simulink model "rocket3"  (R2012b)
settings: Solver=ode3  StartTime=0  StopTime=5  FixedStep=0.0005  RelTol=1e-3
undefined symbols (not defined in the file): dfilt, DiscIntNeverNeededParam, fdesignblkfcn, gcbh
libraries: mblibv1 x17, simulink x1, dsparch4 x1
settings Model: BufferReuse=off  Creator=David  LastModifiedBy=David
settings OptimizationCC: InlineParams=on  BufferReuse=off  SimCompilerOptimization=On
settings DebuggingCC: InitInArrayFormatMsg=none
settings SimMechanicsCC: VisDuringSimulation=on
settings ConfigurationSet: Description=SimMechanics 2G

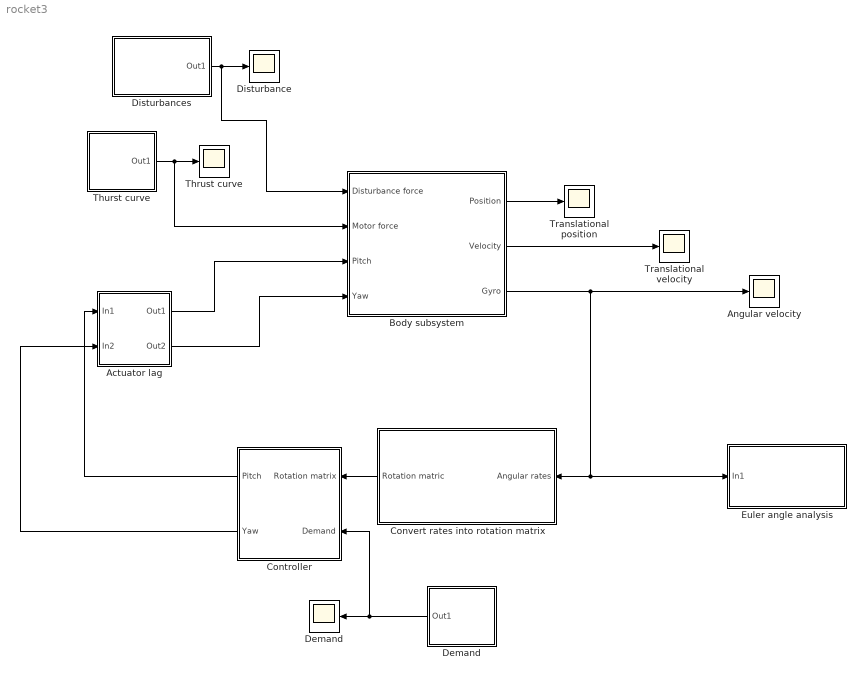
== system rocket3 ==
  Actuator lag : Subsystem
  Angular velocity : Scope
      settings: ShowLegends=on  YMin=-2.5  YMax=0  SaveName=ScopeData2
  Body subsystem : Subsystem
  "Controller " : Subsystem
  Convert rates into rotation matrix : Subsystem
  Demand : Subsystem
  "Demand " : Scope
      settings: YMin=-0.1  YMax=0.09  SaveName=ScopeData8  SampleTime=5
  Disturbance : Scope
      settings: YMin=-0.1  YMax=0.09  SaveName=ScopeData10  SampleTime=5
  Disturbances : Subsystem
  Euler angle analysis : Subsystem
  Thrust curve : Scope
      settings: YMin=-0.1  YMax=0.09  SaveName=ScopeData7
  "Thurst curve " : Subsystem
  Translational position : Scope
      settings: ShowLegends=on
  Translational velocity : Scope
  wires:
  Body subsystem/1(Position) -> Translational position/1
  Body subsystem/2(Velocity) -> Translational velocity/1
  Body subsystem/3(Gyro) -> Angular velocity/1, Euler angle analysis/1(In1), Convert rates into rotation matrix/1(Angular rates)
  Disturbances/1(Out1) -> Body subsystem/1(Disturbance force), Disturbance/1
  "Thurst curve "/1(Out1) -> Body subsystem/2(Motor force), Thrust curve/1
  Convert rates into rotation matrix/1(Rotation matric) -> "Controller "/1(Rotation matrix)
  Demand/1(Out1) -> "Demand "/1, "Controller "/2(Demand)
  "Controller "/1(Pitch) -> Actuator lag/1(In1)
  "Controller "/2(Yaw) -> Actuator lag/2(In2)
  Actuator lag/1(Out1) -> Body subsystem/3(Pitch)
  Actuator lag/2(Out2) -> Body subsystem/4(Yaw)

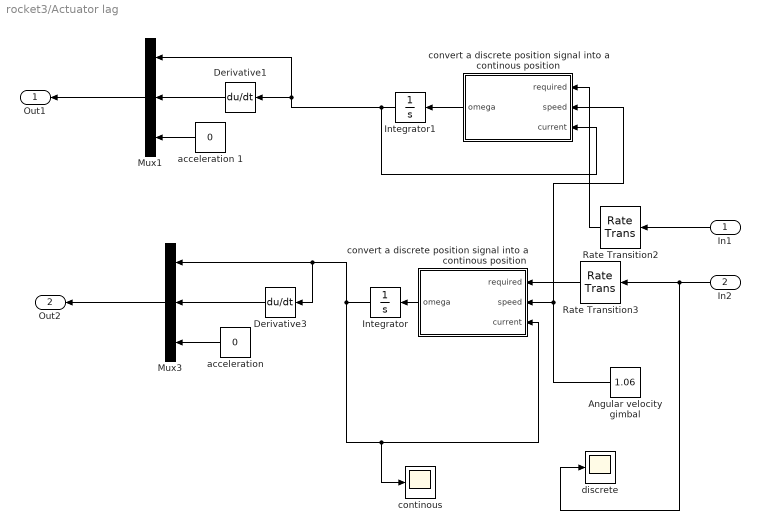
== system rocket3/Actuator lag ==
  In1 : Inport
  In2 : Inport  Port=2
  "Angular velocity gimbal " : Constant  Value=1.06
  Derivative1 : Derivative
  Derivative3 : Derivative
  Integrator : Integrator
  Integrator1 : Integrator
  Mux1 : Mux  Inputs=3
  Mux3 : Mux  Inputs=3
  Rate Transition2 : RateTransition  Deterministic=off  OutPortSampleTimeOpt=Inherit  OutPortSampleTime=0.01
  Rate Transition3 : RateTransition  Deterministic=off  OutPortSampleTimeOpt=Inherit  OutPortSampleTime=0.01
  "acceleration " : Constant  Value=0
  acceleration 1 : Constant  Value=0
  continous : Scope
      settings: TimeRange=5  YMin=-0.06  YMax=0.06  SaveName=ScopeData5
  convert a discrete position signal into a continous position : MATLAB Function  TreatAsAtomicUnit=on
  "convert a discrete position signal into a continous position " : MATLAB Function  TreatAsAtomicUnit=on
  discrete : Scope
      settings: YMin=0.0562129  YMax=0.056213  SaveName=ScopeData4
  Out1 : Outport
  Out2 : Outport  Port=2
  wires:
  In2/1 -> discrete/1, Rate Transition3/1
  In1/1 -> Rate Transition2/1
  "Angular velocity gimbal "/1 -> "convert a discrete position signal into a continous position "/2(speed), convert a discrete position signal into a continous position/2(speed)
  "convert a discrete position signal into a continous position "/1(omega) -> Integrator/1
  Rate Transition3/1 -> "convert a discrete position signal into a continous position "/1(required)
  convert a discrete position signal into a continous position/1(omega) -> Integrator1/1
  Rate Transition2/1 -> convert a discrete position signal into a continous position/1(required)
  Mux3/1 -> Out2/1
  Derivative3/1 -> Mux3/2
  "acceleration "/1 -> Mux3/3
  Integrator/1 -> continous/1, "convert a discrete position signal into a continous position "/3(current), Derivative3/1, Mux3/1
  Mux1/1 -> Out1/1
  Derivative1/1 -> Mux1/2
  acceleration 1/1 -> Mux1/3
  Integrator1/1 -> Mux1/1, Derivative1/1, convert a discrete position signal into a continous position/3(current)

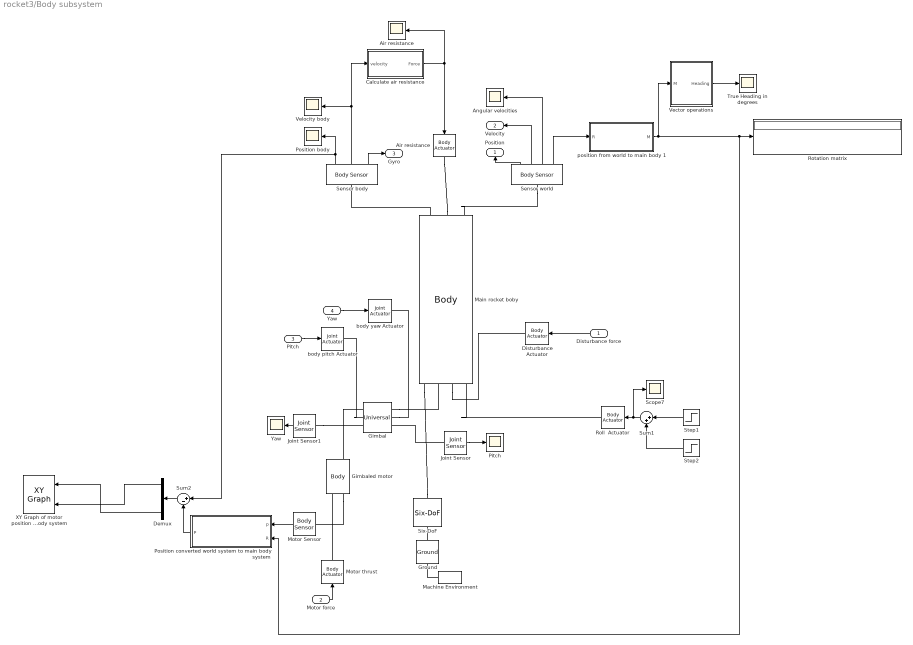
== system rocket3/Body subsystem ==
  Disturbance force : Inport
  Motor force : Inport  Port=2
  Pitch : Inport  Port=3
  Yaw : Inport  Port=4
  Air resistance : mblibv1/Sensors &  Actuators/Body Actuator  UpdateFromCAD=off  PhysicalDomain=Mechanical  PortType=blob  ActuationStyle=Force  AngleUnits=deg  ArcVelocityUnits=deg/s  ArcAccelerationUnits=deg/s^2  CoordPositionUnits=m  VelocityUnits=m/s  AccelerationUnits=m/s^2  ForceUnits=N  TorqueUnits=N*m  ActiveIO=on  Width=3  DialogClass=MechanicalActuatorBlock  ReferenceFrame=Local (Body CS)  Angle=off  CoordPosition=on  Force=on  Torque=off
  "Air resistance " : Scope
      settings: ShowLegends=on  YMin=0  YMax=375  SaveName=ScopeData11
  Angular velocities : Scope
      settings: YMin=0  YMax=375  SaveName=ScopeData20
  Calculate air resistance : MATLAB Function  TreatAsAtomicUnit=on
  Demux : Demux  Outputs=3
  Disturbance Actuator : mblibv1/Sensors &  Actuators/Body Actuator  UpdateFromCAD=off  PhysicalDomain=Mechanical  PortType=blob  ActuationStyle=Force  AngleUnits=deg  ArcVelocityUnits=deg/s  ArcAccelerationUnits=deg/s^2  CoordPositionUnits=m  VelocityUnits=m/s  AccelerationUnits=m/s^2  ForceUnits=N  TorqueUnits=N*m  ActiveIO=on  Width=3  DialogClass=MechanicalActuatorBlock  ReferenceFrame=Local (Body CS)  Angle=off  CoordPosition=on  Force=off  Torque=on
  Gimbal : mblibv1/Joints/Universal  LConnTagsString=__newl0|SA1|SA2  RConnTagsString=__newr0|SA1|SA2  UpdateFromCAD=off  NumSAPorts=4  CutJoint=off  MarkAsCut=off  Primitives=prismatic  PrimitiveProps=R1$Base$[1 0 0]$revolute#R2$Base$[0 0 1]$revolute  DialogClass=JointBlock  R1Axis=[1 0 0]  R2Axis=[0 0 1]
  Gimbaled motor : mblibv1/Bodies/Body  LConnTagsString=CS1|CS2  RConnTagsString=CG|CS3  UpdateFromCAD=off  DialogClass=MechanicalBodyBlock  Mass=0.150  MassUnits=kg  InertiaUnits=g*cm^2  Inertia=[4360 -2 0; -2 194 -11; 0 -11 4363]  Shape=Cylinder  ShapeDims=[1 1]  ShapeUnits=m  ShapeUse=false  Density=1  DensityUnits=kg/m^3  DensityUse=false  GraphicsMode=MACHINE_DEFAULT  BodyColorSelMode=MACHINE_DEFAULT  BodyColor=[1 0 0]  AttachedToCS=CG  CG=Right$CG$[0 -7.4 0]$CS3$CS3$cm$[0 0 0]$Euler X-Y-Z$deg$CS3$true$none  WorkingFrames=Left$CS1$[0 -17 0]$CS3$CS3$cm$[0 0 0]$Euler X-Y-Z$deg$CS3$true$none#Left$CS2$[0 -17 0]$CS3$CS3$cm$[0 0 0]$Euler X-Y-Z$deg$CS3$true$none#Right$CS3$[0 0 0]$Adjoining$Adjoining$cm$[0 0 0]$Euler X-Y-Z$deg$Adjoining$true$none  CGPos=[0 -7.4 0]  CGRot=[0 0 0]  CS0Pos=[]  CS0Rot=[]  CS1Pos=[0 -17 0]  CS1Rot=[0 0 0]  CS2Pos=[0 -17 0]  CS2Rot=[0 0 0]  CS3Pos=[0 0 0]  CS3Rot=[0 0 0]  CS4Pos=[]  CS4Rot=[]  CS5Pos=[]  CS5Rot=[]  CS6Pos=[]  CS6Rot=[]  CS7Pos=[]  CS7Rot=[]  CS8Pos=[]  CS8Rot=[]  CS9Pos=[]  CS9Rot=[]  CS10Pos=[]  CS10Rot=[]  CS11Pos=[]  CS11Rot=[]  CS12Pos=[]  CS12Rot=[]  CS13Pos=[]  CS13Rot=[]  CS14Pos=[]  CS14Rot=[]  CS15Pos=[]  CS15Rot=[]  CS16Pos=[]  CS16Rot=[]  CS17Pos=[]  CS17Rot=[]  CS18Pos=[]  CS18Rot=[]  CS19Pos=[]  CS19Rot=[]  CS20Pos=[]  CS20Rot=[]
  Ground : mblibv1/Bodies/Ground  UpdateFromCAD=off  LeftPortType=env  RightPortType=workingframe  PhysicalDomain=Mechanical  DialogClass=GroundBlock  CoordPosition=[0 0 0]  CoordPositionUnits=m  StateVectorMgrId=-1  MachineId=[0 0]  ShowEnvPort=on
  Joint Sensor : mblibv1/Sensors &  Actuators/Joint Sensor  UpdateFromCAD=off  PhysicalDomain=Mechanical  PortType=blob  Muxed=on  Pose=off  Angle=on  AngleUnits=deg  ArcVelocity=off  ArcVelocityUnits=deg/s  ArcAcceleration=off  ArcAccelerationUnits=deg/s^2  CoordPosition=on  CoordPositionUnits=m  Velocity=off  VelocityUnits=m/s  Acceleration=off  AccelerationUnits=m/s^2  Quaternion=on  QuaternionDT=off  QuaternionDDT=off  QuaternionUnits=off  OutputVector=[1]  ActiveIO=on  Width=1  DialogClass=MechanicalSensorBlock  Primitive=R1  Force=off  ForceUnits=N  Torque=off  TorqueUnits=N*m  ReferenceFrame=Absolute (World)  ReactionSensedSide=Base  ReactionReferenceFrame=Local (Body CS)  ReactionForce=off  ReactionForceUnits=N  ReactionMoment=off  ReactionMomentUnits=N*m
  Joint Sensor1 : mblibv1/Sensors &  Actuators/Joint Sensor  UpdateFromCAD=off  PhysicalDomain=Mechanical  PortType=blob  Muxed=off  Pose=off  Angle=on  AngleUnits=deg  ArcVelocity=off  ArcVelocityUnits=deg/s  ArcAcceleration=off  ArcAccelerationUnits=deg/s^2  CoordPosition=on  CoordPositionUnits=m  Velocity=off  VelocityUnits=m/s  Acceleration=off  AccelerationUnits=m/s^2  Quaternion=on  QuaternionDT=off  QuaternionDDT=off  QuaternionUnits=off  OutputVector=[1]  ActiveIO=on  Width=1  DialogClass=MechanicalSensorBlock  Primitive=R2  Force=off  ForceUnits=N  Torque=off  TorqueUnits=N*m  ReferenceFrame=Absolute (World)  ReactionSensedSide=Base  ReactionReferenceFrame=Local (Body CS)  ReactionForce=off  ReactionForceUnits=N  ReactionMoment=off  ReactionMomentUnits=N*m
  Machine Environment : mblibv1/Bodies/Machine Environment  PortType=env  PhysicalDomain=Mechanical  DialogTemplateClass=MECH.MachineEnvironment  SyncWhenCopied=off  Gravity=[0 -9.81 0]  GravityUnits=m/s^2  GravityAsSignal=off  Dimensionality=Auto-detect  AnalysisType=Forward dynamics  LinearAssemblyTolerance=1e-3  LinearAssemblyToleranceUnits=m  AngularAssemblyTolerance=1e-3  AngularAssemblyToleranceUnits=rad  ConstraintSolverType=Stabilizing  ConstraintRelTolerance=1e-4  ConstraintAbsTolerance=1e-4  UseRobustSingularityHandling=off  RedundancyAnalysisToleranceType=Automatically select tolerance  RedundancyAnalysisTolerance=1e-14  StatePerturbationType=Fixed  PerturbationSize=1e-5  VisualizeMachine=on  BodyVisualizationType=Use model default body geometries  BodyColorSelMode=Use model default  DefaultBodyColor=[1 0 0]
  Main rocket boby : mblibv1/Bodies/Body  LConnTagsString=CG|CS5|CS1|CS6  RConnTagsString=CS3|CS2|CS4  UpdateFromCAD=off  DialogClass=MechanicalBodyBlock  Mass=1  MassUnits=kg  InertiaUnits=g*cm^2  Inertia=[433353 -160 147; -160 9482 62; 147 62 433391]  Shape=Cylinder  ShapeDims=[1 1]  ShapeUnits=m  ShapeUse=false  Density=1  DensityUnits=kg/m^3  DensityUse=false  GraphicsMode=MACHINE_DEFAULT  BodyColorSelMode=MACHINE_DEFAULT  BodyColor=[1 0 0]  AttachedToCS=CG  CG=Left$CG$[0 39.4 0]$WORLD$WORLD$cm$[0 0 0]$Euler X-Y-Z$deg$World$true$none  WorkingFrames=Left$CS5$[0 -21.6 0]$CG$CG$cm$[0 0 0]$Euler X-Y-Z$deg$CG$true$none#Left$CS1$[0 5 0]$CG$CG$cm$[0 0 0]$Euler X-Y-Z$deg$CG$true$none#Right$CS3$[0 0 0]$CG$CG$cm$[0 0 0]$Euler X-Y-Z$deg$CG$true$none#Right$CS2$[0 30 0]$CG$CG$cm$[0 0 0]$Euler X-Y-Z$deg$CG$true$none#Right$CS4$[0 0 0]$CG$CG$cm$[0 0 0]$Euler X-Y-Z$deg$CG$true$none#Left$CS6$[0 0 0]$CG$CG$cm$[0 0 0]$Euler X-Y-Z$deg$CG$true$none  CGPos=[0 39.4 0]  CGRot=[0 0 0]  CS0Pos=[]  CS0Rot=[]  CS1Pos=[0 5 0]  CS1Rot=[0 0 0]  CS2Pos=[0 30 0]  CS2Rot=[0 0 0]  CS3Pos=[0 0 0]  CS3Rot=[0 0 0]  CS4Pos=[0 0 0]  CS4Rot=[0 0 0]  CS5Pos=[0 -21.6 0]  CS5Rot=[0 0 0]  CS6Pos=[0 0 0]  CS6Rot=[0 0 0]  CS7Pos=[]  CS7Rot=[]  CS8Pos=[]  CS8Rot=[]  CS9Pos=[]  CS9Rot=[]  CS10Pos=[]  CS10Rot=[]  CS11Pos=[]  CS11Rot=[]  CS12Pos=[]  CS12Rot=[]  CS13Pos=[]  CS13Rot=[]  CS14Pos=[]  CS14Rot=[]  CS15Pos=[]  CS15Rot=[]  CS16Pos=[]  CS16Rot=[]  CS17Pos=[]  CS17Rot=[]  CS18Pos=[]  CS18Rot=[]  CS19Pos=[]  CS19Rot=[]  CS20Pos=[]  CS20Rot=[]
  Motor Sensor : mblibv1/Sensors &  Actuators/Body Sensor  UpdateFromCAD=off  PhysicalDomain=Mechanical  PortType=blob  Muxed=off  Pose=off  Angle=on  AngleUnits=deg  ArcVelocity=off  ArcVelocityUnits=deg/s  ArcAcceleration=off  ArcAccelerationUnits=deg/s^2  CoordPosition=on  CoordPositionUnits=m  Velocity=off  VelocityUnits=m/s  Acceleration=off  AccelerationUnits=m/s^2  Quaternion=on  QuaternionDT=off  QuaternionDDT=off  QuaternionUnits=off  OutputVector=[1]  ActiveIO=on  Width=3  DialogClass=MechanicalSensorBlock  ReferenceFrame=Absolute (World)
  Motor thrust : mblibv1/Sensors &  Actuators/Body Actuator  UpdateFromCAD=off  PhysicalDomain=Mechanical  PortType=blob  ActuationStyle=Force  AngleUnits=deg  ArcVelocityUnits=deg/s  ArcAccelerationUnits=deg/s^2  CoordPositionUnits=m  VelocityUnits=m/s  AccelerationUnits=m/s^2  ForceUnits=N  TorqueUnits=N*m  ActiveIO=on  Width=3  DialogClass=MechanicalActuatorBlock  ReferenceFrame=Local (Body CS)  Angle=off  CoordPosition=on  Force=on  Torque=off
  "Pitch " : Scope
      settings: SaveName=ScopeData9
  Position body : Scope
      settings: YMin=0  YMax=375  SaveName=ScopeData22
  "Position converted world system to main body system " : MATLAB Function  TreatAsAtomicUnit=on
  Roll  Actuator : mblibv1/Sensors &  Actuators/Body Actuator  UpdateFromCAD=off  PhysicalDomain=Mechanical  PortType=blob  ActuationStyle=Force  AngleUnits=deg  ArcVelocityUnits=deg/s  ArcAccelerationUnits=deg/s^2  CoordPositionUnits=m  VelocityUnits=m/s  AccelerationUnits=m/s^2  ForceUnits=N  TorqueUnits=N*m  ActiveIO=on  Width=3  DialogClass=MechanicalActuatorBlock  ReferenceFrame=Local (Body CS)  Angle=off  CoordPosition=on  Force=off  Torque=on
  Rotation matrix : Display
  Scope7 : Scope
      settings: ShowLegends=on  YMin=0  YMax=375  SaveName=ScopeData27
  Sensor body : mblibv1/Sensors &  Actuators/Body Sensor  UpdateFromCAD=off  PhysicalDomain=Mechanical  PortType=blob  Muxed=off  Pose=off  Angle=on  AngleUnits=deg  ArcVelocity=on  ArcVelocityUnits=rad/s  ArcAcceleration=off  ArcAccelerationUnits=deg/s^2  CoordPosition=on  CoordPositionUnits=m  Velocity=on  VelocityUnits=m/s  Acceleration=off  AccelerationUnits=m/s^2  Quaternion=on  QuaternionDT=off  QuaternionDDT=off  QuaternionUnits=off  OutputVector=[1]  ActiveIO=on  Width=9  DialogClass=MechanicalSensorBlock  ReferenceFrame=Local (Body CS)
  Sensor world : mblibv1/Sensors &  Actuators/Body Sensor  UpdateFromCAD=off  PhysicalDomain=Mechanical  PortType=blob  Muxed=off  Pose=on  Angle=on  AngleUnits=deg  ArcVelocity=on  ArcVelocityUnits=rad/s  ArcAcceleration=off  ArcAccelerationUnits=deg/s^2  CoordPosition=on  CoordPositionUnits=m  Velocity=on  VelocityUnits=m/s  Acceleration=off  AccelerationUnits=m/s^2  Quaternion=on  QuaternionDT=off  QuaternionDDT=off  QuaternionUnits=off  OutputVector=[1]  ActiveIO=on  Width=18  DialogClass=MechanicalSensorBlock  ReferenceFrame=Absolute (World)
  Six-DoF : mblibv1/Joints/Six-DoF  LConnTagsString=__newl0  RConnTagsString=__newr0  UpdateFromCAD=off  NumSAPorts=0  CutJoint=off  MarkAsCut=off  Primitives=prismatic_prismatic  PrimitiveProps=P1$World$[1 0 0]$prismatic#P2$World$[0 1 0]$prismatic#P3$World$[0 0 1]$prismatic#S$World$[0 0 0]$spherical  DialogClass=JointBlock  P1Axis=[1 0 0]  P2Axis=[0 1 0]  P3Axis=[0 0 1]  SAxis=[0 0 0]
  Step1 : Step  Time=[2,1,2]  Before=[0,0,0]  After=[0,0,0]  SampleTime=0  VectorParams1D=off
  Step2 : Step  Time=[2.0,1.01, 2.0]  Before=[0,0,0]  After=[0,0, 0]  SampleTime=0  VectorParams1D=off
  Sum1 : Sum  Inputs=|++
  Sum2 : Sum  Inputs=|+-
  True Heading in degrees : Scope
      settings: YMin=0.99675  YMax=1.00025  SaveName=ScopeData26
  Vector operations : MATLAB Function  TreatAsAtomicUnit=on
  Velocity body : Scope
      settings: ShowLegends=on  YMin=0  YMax=375  SaveName=ScopeData21
  XY Graph of motor position relative to body system : simulink/Sinks/XY Graph  xmin=-0.02  xmax=0.02  ymin=-0.02  ymax=0.02  st=-1
  "Yaw " : Scope
      settings: SaveName=ScopeData14
  body pitch Actuator : mblibv1/Sensors &  Actuators/Joint Actuator  UpdateFromCAD=off  PhysicalDomain=Mechanical  PortType=blob  ActuationStyle=Motion  AngleUnits=rad  ArcVelocityUnits=rad/s  ArcAccelerationUnits=rad/s^2  CoordPositionUnits=m  VelocityUnits=m/s  AccelerationUnits=m/s^2  ForceUnits=N  TorqueUnits=N*m  ActiveIO=on  Width=3  DialogClass=MechanicalActuatorBlock  Primitive=R1  ReferenceFrame=Absolute (World)
  body yaw Actuator : mblibv1/Sensors &  Actuators/Joint Actuator  UpdateFromCAD=off  PhysicalDomain=Mechanical  PortType=blob  ActuationStyle=Motion  AngleUnits=rad  ArcVelocityUnits=rad/s  ArcAccelerationUnits=rad/s^2  CoordPositionUnits=m  VelocityUnits=m/s  AccelerationUnits=m/s^2  ForceUnits=N  TorqueUnits=N*m  ActiveIO=on  Width=3  DialogClass=MechanicalActuatorBlock  Primitive=R2  ReferenceFrame=Absolute (World)
  position from world to main body 1 : MATLAB Function  TreatAsAtomicUnit=on
  Position : Outport
  Velocity : Outport  Port=2
  Gyro : Outport  Port=3
  wires:
  Sensor body/1 -> Sum2/1, Position body/1
  Disturbance force/1 -> Disturbance Actuator/1
  Sensor body/3 -> Gyro/1
  Joint Sensor/1 -> "Pitch "/1
  Sensor body/2 -> Calculate air resistance/1(velocity), Velocity body/1
  Joint Sensor1/1 -> "Yaw "/1
  Sensor world/3 -> Angular velocities/1
  Step1/1 -> Sum1/1
  Step2/1 -> Sum1/2
  Sum1/1 -> Scope7/1, Roll  Actuator/1
  Sensor world/2 -> Velocity/1
  Demux/1 -> XY Graph of motor position relative to body system/2
  Demux/3 -> XY Graph of motor position relative to body system/1
  Sum2/1 -> Demux/1
  Sensor world/1 -> Position/1
  Motor Sensor/1 -> "Position converted world system to main body system "/1(p)
  "Position converted world system to main body system "/1(P) -> Sum2/2
  Sensor world/4 -> position from world to main body 1/1(R)
  position from world to main body 1/1(M) -> Rotation matrix/1, "Position converted world system to main body system "/2(R), Vector operations/1(M)
  Vector operations/1(Heading) -> True Heading in degrees/1
  Motor force/1 -> Motor thrust/1
  Calculate air resistance/1(Force) -> Air resistance/1, "Air resistance "/1
  Yaw/1 -> body yaw Actuator/1
  Pitch/1 -> body pitch Actuator/1
  connections:
  Main rocket boby/LConn3 -- Disturbance Actuator/RConn1
  Motor thrust/RConn1 -- Gimbaled motor/LConn1
  Ground/RConn1 -- Six-DoF/LConn1
  Machine Environment/RConn1 -- Ground/LConn1
  Main rocket boby/RConn1 -- Sensor body/LConn1
  Main rocket boby/LConn1 -- Six-DoF/RConn1
  Gimbal/LConn1 -- Main rocket boby/LConn2
  Gimbal/RConn2 -- body pitch Actuator/RConn1
  Gimbal/LConn2 -- body yaw Actuator/RConn1
  Gimbaled motor/RConn2 -- Gimbal/RConn1
  Gimbaled motor/LConn2 -- Motor Sensor/LConn1
  Joint Sensor/LConn1 -- Gimbal/LConn3
  Air resistance/RConn1 -- Main rocket boby/RConn2
  Joint Sensor1/LConn1 -- Gimbal/RConn3
  Sensor world/LConn1 -- Main rocket boby/RConn3
  Roll  Actuator/RConn1 -- Main rocket boby/LConn4

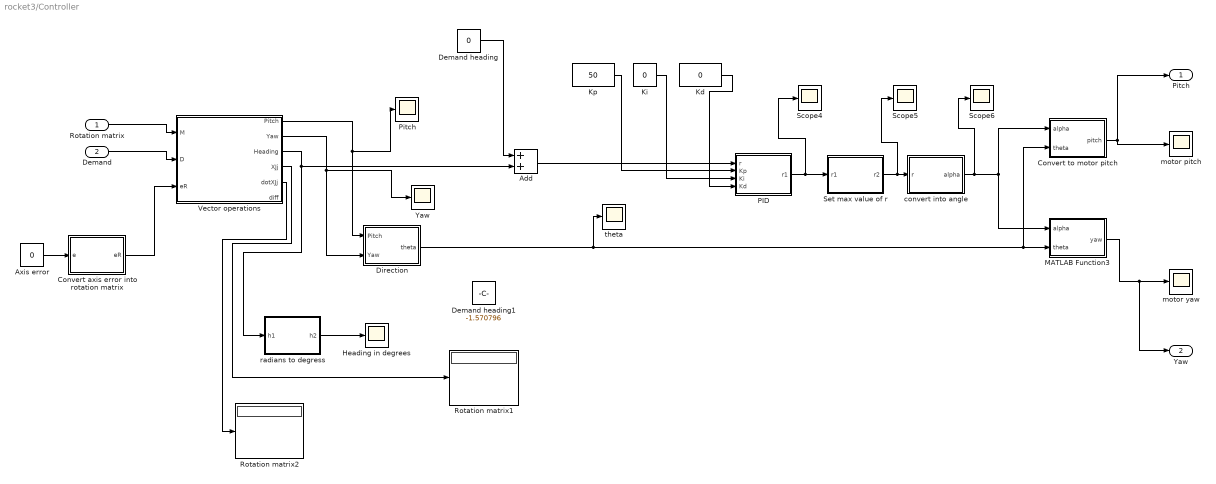
== system rocket3/Controller  ==
  Rotation matrix : Inport
  Demand : Inport  Port=2
  " Direction" : MATLAB Function  TreatAsAtomicUnit=on
  " PID" : MATLAB Function  TreatAsAtomicUnit=on
  Add : Sum
  Axis error : Constant  Value=0
  Convert axis error into rotation matrix : MATLAB Function  TreatAsAtomicUnit=on
  Convert to motor pitch : MATLAB Function  TreatAsAtomicUnit=on
  Demand heading : Constant  Value=0
  Demand heading1 : Constant  Value=-1.570796
  Heading in degrees : Scope
      settings: TimeRange=5  YMin=-1.5  YMax=7.5  SaveName=ScopeData6
  Kd : Constant  Value=0  SampleTime=0.01
  Ki : Constant  Value=0  SampleTime=0.01
  Kp : Constant  Value=50  SampleTime=0.01
  MATLAB Function3 : MATLAB Function  TreatAsAtomicUnit=on
  "Pitch " : Scope
      settings: YMin=-0.375  YMax=-0.345  SaveName=ScopeData29
  Rotation matrix1 : Display
  Rotation matrix2 : Display
  Scope4 : Scope
      settings: YMin=1  YMax=16  SaveName=ScopeData16
  Scope5 : Scope
      settings: YMin=9.025  YMax=9.975  SaveName=ScopeData17
  Scope6 : Scope
      settings: SaveName=ScopeData18
  Set max value of r : MATLAB Function  TreatAsAtomicUnit=on
  Vector operations : MATLAB Function  TreatAsAtomicUnit=on
  "Yaw " : Scope
      settings: YMin=0.625  YMax=0.71  SaveName=ScopeData30
  convert into angle : MATLAB Function  TreatAsAtomicUnit=on
  motor pitch : Scope
      settings: SaveName=ScopeData24
  motor yaw : Scope
      settings: SaveName=ScopeData25
  "radians to degress " : MATLAB Function  TreatAsAtomicUnit=on
  theta : Scope
      settings: YMin=-3  YMax=1.25  SaveName=ScopeData31
  Pitch : Outport
  Yaw : Outport  Port=2
  wires:
  Set max value of r/1(r2) -> Scope5/1, convert into angle/1(r)
  convert into angle/1(alpha) -> Scope6/1, Convert to motor pitch/1(alpha), MATLAB Function3/1(alpha)
  Convert to motor pitch/1(pitch) -> Pitch/1, motor pitch/1
  MATLAB Function3/1(yaw) -> Yaw/1, motor yaw/1
  " PID"/1(r1) -> Scope4/1, Set max value of r/1(r1)
  Kp/1 -> " PID"/2(Kp)
  Ki/1 -> " PID"/3(Ki)
  Kd/1 -> " PID"/4(Kd)
  Rotation matrix/1 -> Vector operations/1(M)
  Vector operations/1(Pitch) -> " Direction"/1(Pitch), "Pitch "/1
  Vector operations/2(Yaw) -> "Yaw "/1, " Direction"/2(Yaw)
  " Direction"/1(theta) -> theta/1, Convert to motor pitch/2(theta), MATLAB Function3/2(theta)
  Vector operations/3(Heading) -> Add/2, "radians to degress "/1(h1)
  "radians to degress "/1(h2) -> Heading in degrees/1
  Demand/1 -> Vector operations/2(D)
  Axis error/1 -> Convert axis error into rotation matrix/1(e)
  Convert axis error into rotation matrix/1(eR) -> Vector operations/3(eR)
  Add/1 -> " PID"/1(r)
  Demand heading/1 -> Add/1
  Vector operations/4(XJj) -> Rotation matrix1/1
  Vector operations/5(dotXJj) -> Rotation matrix2/1

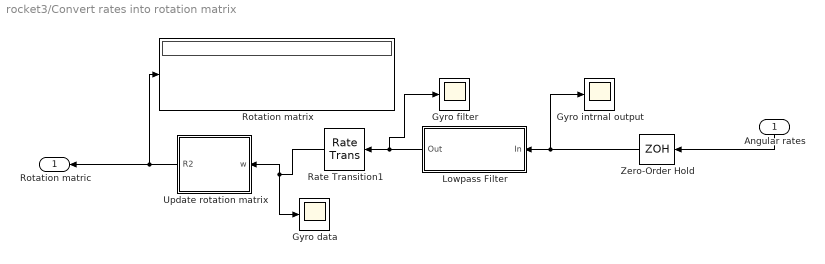
== system rocket3/Convert rates into rotation matrix ==
  Angular rates : Inport
  Gyro data : Scope
      settings: ShowLegends=on  SaveName=ScopeData19
  Gyro filter : Scope
      settings: ShowLegends=on  SaveName=ScopeData13
  Gyro intrnal output : Scope
      settings: ShowLegends=on  SaveName=ScopeData23
  Lowpass Filter : Subsystem  DialogController=fdesignblkfcn  InitFcn=fdesignblkfcn(gcbh, {'InitFcn'});  mask(Lowpass Filter){}
      mask help: Design a lowpass filter
      settings: CopyFcn=fdesignblkfcn(gcbh, {'CopyFcn'});
      mask Help: helpview(mapfilelocation('dsp'), 'dsplowpassfilter');
      mask Display: disp('Lowpass')
  Rate Transition1 : RateTransition  Deterministic=off  OutPortSampleTime=0.01
  Rotation matrix : Display
  Update rotation matrix : MATLAB Function  TreatAsAtomicUnit=on
  Zero-Order Hold : ZeroOrderHold  SampleTime=0.001
  Rotation matric : Outport
  wires:
  Angular rates/1 -> Zero-Order Hold/1
  Update rotation matrix/1(R2) -> Rotation matric/1, Rotation matrix/1
  Zero-Order Hold/1 -> Gyro intrnal output/1, Lowpass Filter/1(In)
  Lowpass Filter/1(Out) -> Gyro filter/1, Rate Transition1/1
  Rate Transition1/1 -> Gyro data/1, Update rotation matrix/1(w)

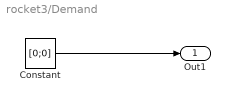
== system rocket3/Demand ==
  Constant : Constant  Value=[0;0]
  Out1 : Outport
  wires:
  Constant/1 -> Out1/1

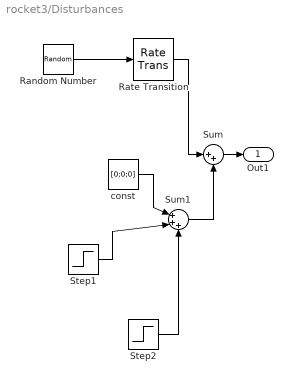
== system rocket3/Disturbances ==
  Random Number : RandomNumber  Mean=[0.0;0;0]  Variance=[0;0;0]  SampleTime=0.001  VectorParams1D=off
  Rate Transition : RateTransition  Deterministic=off  OutPortSampleTimeOpt=Inherit
  Step1 : Step  Time=[0.5;0.5;0.5]  Before=[0;0;0]  After=[2;2;2]  SampleTime=0  VectorParams1D=off
  Step2 : Step  Time=[0.51;0.5;0.50]  Before=[0;0;0]  After=[-2;-2;-2]  SampleTime=0  VectorParams1D=off
  Sum : Sum  Inputs=|++
  Sum1 : Sum  Inputs=|+++
  const : Constant  Value=[0;0;0]  VectorParams1D=off
  Out1 : Outport
  wires:
  Sum/1 -> Out1/1
  Sum1/1 -> Sum/2
  const/1 -> Sum1/1
  Step1/1 -> Sum1/2
  Step2/1 -> Sum1/3
  Random Number/1 -> Rate Transition/1
  Rate Transition/1 -> Sum/1

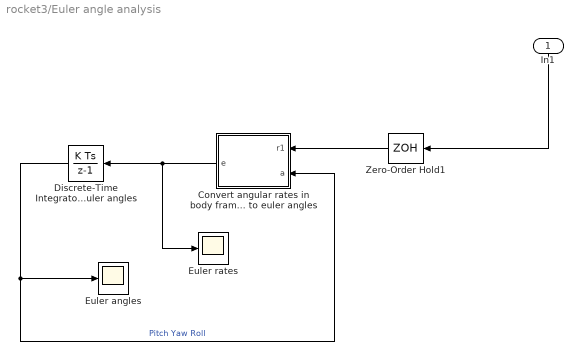
== system rocket3/Euler angle analysis ==
  In1 : Inport
  Convert angular rates in body frame to euler angles : MATLAB Function  TreatAsAtomicUnit=on
  Discrete-Time Integrator for euler angles : DiscreteIntegrator  gainval=1  SampleTime=0.01  ICPrevOutput=DiscIntNeverNeededParam  ICPrevScaledInput=DiscIntNeverNeededParam
  Euler angles : Scope
      settings: ShowLegends=on  YMin=0.05  YMax=0.9  SaveName=ScopeData3
  "Euler rates " : Scope
      settings: ShowLegends=on  SaveName=ScopeData28
  Zero-Order Hold1 : ZeroOrderHold  SampleTime=0.01
  wires:
  In1/1 -> Zero-Order Hold1/1
  Discrete-Time Integrator for euler angles/1 -> Euler angles/1, Convert angular rates in body frame to euler angles/2(a)  "Pitch Yaw Roll"
  Convert angular rates in body frame to euler angles/1(e) -> "Euler rates "/1, Discrete-Time Integrator for euler angles/1
  Zero-Order Hold1/1 -> Convert angular rates in body frame to euler angles/1(r1)

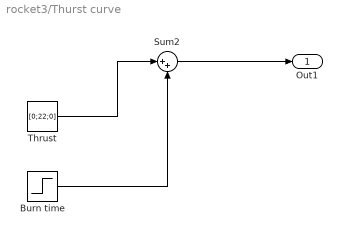
== system rocket3/Thurst curve  ==
  Burn time : Step  Time=[0;5; 0]  Before=[0;0;0]  After=[0;0;0]  SampleTime=0  VectorParams1D=off
  Sum2 : Sum  Inputs=|++
  Thrust : Constant  Value=[0;22;0]  VectorParams1D=off
  Out1 : Outport
  wires:
  Thrust/1 -> Sum2/1
  Sum2/1 -> Out1/1
  Burn time/1 -> Sum2/2

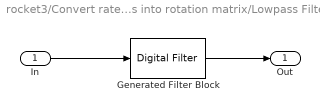
== system rocket3/Convert rates into rotation matrix/Lowpass Filter ==
  In : Inport
  Generated Filter Block : dsparch4/Digital Filter  Tag=BlockMethodSubSystem  TypePopup=FIR (all zeros)  IIRFiltStruct=Direct form II transposed  AllPoleFiltStruct=Direct form  FIRFiltStruct=Direct form  CoeffSource=Specify via dialog  NumCoeffs=[-0.0086576118436237099 -0.029483359899297831 -0.031006311548444312 0.043288171023261351 0.1964326006000513 0.33033263240797889 0.33033263240797889 0.1964326006000513 0.043288171023261351 -0.031006311548444312 -0.029483359899297831 -0.0086576118436237099]  DenCoeffs=[1 0.1]  BiQuadCoeffs=[1 0.3 0.4 1 0.1 0.2]  LatticeCoeffs=[0.2 0.4]  denIgnore=on  FiltPerSampPopup=One filter per frame  IC=0  ICnum=0  ICden=0  roundingMode=Floor  overflowMode=off  ScaleValues=1  scaleValueFracLength=14  stageInFracLength=15  stageOutFracLength=15  FilterSource=Specify via dialog  dfiltObjectName=dfilt.dffir([1 2 1])
  Out : Outport
  wires:
  In/1 -> Generated Filter Block/1
  Generated Filter Block/1 -> Out/1

== matlab function rocket3/Body subsystem/Position converted world system to main body system  ==
  data: p input; R input; P output
function P = fcn(p, R)
%#codegen

    R = inv(R);

    P = R * p;
end

== matlab function rocket3/Body subsystem/Calculate air resistance ==
  data: velocity input; Force output
function Force = fcn(velocity)
%#codegen
air_density = 1.25;
frontal_area = 0.084^2 * pi / 4;
%side_area =
front_coef = 1; %currently a complete guess 
%side_coef =
Force = zeros(3,1);
%Force(1) = 0.5*side_area * side_coef * air_density*velocity(1)^2;
Force(2) = -0.5 * frontal_area * front_coef * air_density*velocity(2)^2;
%Force(3) = 0.5*side_area * side_coef * air_density*velocity(1)^2;
Force(1) = 0;
Force(3) = 0;
end

== matlab function rocket3/Controller /radians to degress  ==
  data: h1 input; h2 output
function h2 = fcn(h1)
%#codegen
h2 = h1*180/pi;
end

== matlab function rocket3/Body subsystem/position from world to main body 1 ==
  data: R input; M output
function M = fcn(R)
%#codegen

    M=zeros(3,3); %so R is matrix but isn't wtf matlab
    M(1,1)= R(1);
    M(2,1)= R(2);
    M(3,1)= R(3);
    M(1,2)= R(4);
    M(2,2)= R(5);
    M(3,2)= R(6);
    M(1,3)= R(7);
    M(2,3)= R(8);
    M(3,3)= R(9);
    
end

== matlab function rocket3/Controller /Convert axis error into rotation matrix ==
  data: e input; eR output
function eR = fcn(e)
%convert error into radians of rotation
error=e*2*pi();

R1=[1 0 0
    0 cos(error) -sin(error)
    0 sin(error) cos(error)];

R2=[cos(error) 0 sin(error)
    0 1 0
    -sin(error) 0 cos(error)];

R3=[cos(error) -sin(error) 0
    sin(error) cos(error) 0
    0 0 1];

eR=R3*R2*R1;
end

== matlab function rocket3/Body subsystem/Vector operations ==
  data: M input; Heading output
function Heading  = fcn(M)
%#codegen
%unit vectors in the inertial frame
I = [1 %in X direction
     0 
     0];
J = [0 %in Y direction
     1
     0];
K = [0 %in Z direction
     0
     1];
%the matrix is composed of the unit vectors aligned with the body
%coordinate system
i = M(:,1); %in x direction
j = M(:,2); %in y direction
k = M(:,3); %in z direction

%take dot product


Heading = acos( dot(j,J)/(norm(J)*norm(j)) );
Heading = Heading*180/pi;

end

== matlab function rocket3/Actuator lag/convert a discrete position signal into a continous position  ==
  data: required input; omega output; speed input; current input
function omega = fcn(required, speed, current)
if current <= required
    omega = speed;
else
    omega = -speed;
end

if current == required
    omega = 0;
end

end

== matlab function rocket3/Actuator lag/convert a discrete position signal into a continous position ==
  data: required input; omega output; speed input; current input
function omega = fcn(required, speed, current)
if current <= required
    omega = speed;
else
    omega = -speed;
end

if current == required
    omega = 0;
end

end

== matlab function rocket3/Euler angle analysis/Convert angular rates in body frame to euler angles ==
  data: r1 input; e output; a input size=3
function e = fcn(r1, a)
    %{
    Note: Euler angle convention PITCH, YAW, ROLL (in that order) where:
    Pitch is rotation about the x axis of the rocket (when initially
    aligned with the inertial frame
    Yaw is a rotation about z axis of the rocket after pitch
    Roll is rotation about the y axis of the rocket after yaw
    These are intrinsic tait-bryan angles (x, z', y'').
    Extrinsic angles are measured about the Y Z X axis (in that order), 
    with the angles being ROLL, YAW, PITCH (that order) 
    Note 2: the above definitions are different to those commonly used for
    aeroplanes
    
    
    r1(1) is rate of rotation about the rocket's x axis 
    r1(2) is rate of rotation about the rocket's y axis
    r1(3) is rate of rotation about the rocket's z axis
    r2(1) is rate of rotation about the rocket's x axis 
    r2(2) is rate of rotation about the rocket's z axis
    r2(3) is rate of rotation about the rocket's y axis
    a(1) is PITCH
    a(2) is YAW
    a(3) is ROLL
    e(1) is pitch rate
    e(2) is yaw rate
    e(3) is roll rate
    %}

%{
e = [r(2) + r(1) * sin(a(1)) * tan(a(2)) + r(3) * cos(a(1)) * tan( a(2))
     r(1) * cos(a(1)) - r(3) * sin(a(1))
     r(1) * sin(a(1))/cos(a(2)) + r(3) * cos(a(1))/cos(a(2)) ];
%}
r2 = [  r1(1)
        r1(3)
        r1(2)];
  
   R = [cos(a(3))/cos(a(2))      sin(a(3))/cos(a(2))       0
        -sin(a(3))               cos(a(3))                 0
        cos(a(3)) * tan( a(2))   sin(a(3)) * tan(a(2))     1  ];
 
  e = R * r2;
end

== matlab function rocket3/Controller /Vector operations ==
  data: M input; Pitch output; Yaw output; Heading output; D input; eR input; XJj output; dotXJj output; diff output
function [Pitch,Yaw,Heading, XJj, dotXJj, diff] = fcn(M, D, eR)
%#codegen
%unit vectors in the inertial frame
I = [1 %in X direction
     0 
     0];
J = [0 %in Y direction
     1
     0];
K = [0 %in Z direction
     0
     1];
 
%the default demand is to head in the directions of J
%the demand is a 2D vector containing the containing alpha and beta (think spherical coords)
%for the unit vector we want to go in, alpha being the angle 
%convert demand from ° to rads
D=D*pi()/180;
%find new J
J=[sin(D(2)) * cos(D(1)) 
   cos(D(2))
   sin(D(2)) * sin(D(1))];

%directions
%the matrix is composed of the unit vectors aligned with the body
%if the axis of the sensor are not aligned with the axis of the gimbal
%there will be an error
M=M*eR;
%coordinate system
i = M(:,1); %in x direction
j = M(:,2); %in y direction
k = M(:,3); %in z direction

%take dot products
%{
Pitch is rotation about the x axis of the rocket (when initially
aligned with the inertial frame
Yaw is a rotation about z axis of the rocket after pitch
Roll is rotation about the y axis of the rocket after yaw
%}
    
Pitch = asin( dot(k,J)/(norm(J)*norm(k)) ); %this gives the angle between the z axis and the
                           % horizontal plan (in which I and K reside)
                           %when no pitch is required this angle will be 0
Yaw = asin ( dot(i,J)/(norm(J)*norm(i)) );


Heading = acos( dot(j,J)/(norm(J)*norm(j)) );

%need to determine if heading should be negative to allow the PID to do
%its job, when the cross product suddenly changes direction the heading
%should change sign
XJj=cross(J,j);
XJj=XJj/norm(XJj);
persistent pre_XJj flip_coefficient;
if isempty(pre_XJj) 
    pre_XJj=cross(J,j);
    flip_coefficient = 1;
end

if dot(XJj, pre_XJj) < 0
    flip_coefficient =-1*flip_coefficient;
end

dotXJj=dot(XJj, pre_XJj)
diff =XJj-pre_XJj;
Heading = Heading * flip_coefficient;
pre_XJj=XJj;

end

== matlab function rocket3/Controller /Convert to motor pitch ==
  data: alpha input; pitch output; theta input
function pitch = fcn(alpha, theta)
%#codegen
pitch = - alpha * cos(theta);  
end

== matlab function rocket3/Controller /MATLAB Function3 ==
  data: alpha input; yaw output; theta input
function yaw = fcn(alpha, theta)
%#codegen
yaw = - alpha * sin(theta);

== matlab function rocket3/Controller / PID ==
  data: r input; r1 output; Kp input; Ki input; Kd input
function r1 = fcn(r, Kp, Ki, Kd)

%#codegen
%Kp = 0;
%Ki = 0;
%Kd = 0;
time_step = 0.01;
persistent Integral previous_r  Der Der_pre;
if isempty(previous_r) 
    Integral = 0;
    Der = 0;
    Der_pre =0;
    previous_r = r;
    i=0;
end

    if (previous_r < 10) %stop integral causing windup
        Integral = Integral + r * time_step;
    end
    Der = (r - previous_r)/ time_step;
    previous_r = r;
    %filter the Der
    a = 0.9;
    Der = (1 -a) * Der + a * Der_pre; % 0 < a < 1
    Der_pre = Der;
    
    r1 = Kp * r + Ki*Integral + Kd * Der;
   
end

== matlab function rocket3/Controller /Set max value of r ==
  data: r1 input; r2 output
function r2 = fcn(r1)
%#codegen
r2 = abs(r1); %remove negative as the angle is set independently
if r1 > 9.5
    r2 = 9.5;
end

== matlab function rocket3/Controller /convert into angle ==
  data: r input; alpha output
function alpha = fcn(r)
%#codegen 
a = 164 + 5;
alpha = r / a;
end

== matlab function rocket3/Convert rates into rotation matrix/Update rotation matrix ==
  data: w input; R2 output
function R2 = fcn(w)
%{
R1 is the previous rotation matrix which rotates the inertial 
coordinate system to the body one
R2 is the new matrix updated with the rotation rates from the body frame
w is the rotation vector for the body frame 
w(1) is rate of rotation about the rocket's x axis 
w(2) is rate of rotation about the rocket's y axis
w(3) is rate of rotation about the rocket's z axis
%}



delta_t = 0.01;

persistent  R1;
if isempty(R1) 
    R1 = eye(3);
end

R2 = R1 * [ 1             -w(3)*delta_t  w(2)*delta_t
            w(3)*delta_t  1              -w(1)*delta_t
            -w(2)*delta_t w(1)*delta_t   1              ];

%Renormalization of R
xy_error=dot(R2(:,1),R2(:,2));
R3=zeros(3,3);
R3(:,1) = R2(:,1) - 0.5*xy_error*R2(:,2);
R3(:,2) = R2(:,2) - 0.5*xy_error*R2(:,1);
R3(:,3) = cross(R3(:,1),R3(:,2));
%make magnitudes equal to one, as the difference will be small can use
%taylor expansion to avoid square root
R3(:,1) = 0.5*(3 - dot(R3(:,1),R3(:,1))) * R3(:,1);
R3(:,2) = 0.5*(3 - dot(R3(:,2),R3(:,2))) * R3(:,2);
R3(:,3) = 0.5*(3 - dot(R3(:,3),R3(:,3))) * R3(:,3);

R1 = R3; 

end

== matlab function rocket3/Controller / Direction ==
  data: Pitch input; Yaw input; theta output
function theta = fcn(Pitch, Yaw)
%#codegen
if Pitch == 0
    Pitch = 0.00000;
end

theta = - atan2(Yaw,Pitch); % minus signs may need to be added to make sure theta acts in the direction to conteract the rotation
